simulink model "Basic_LogicGates"  (R2018a)
settings: Solver=VariableStepAuto  StartTime=0.0  StopTime=10.0  RelTol=1e-3
settings Model: Creator=Asus  LastModifiedBy=Asus

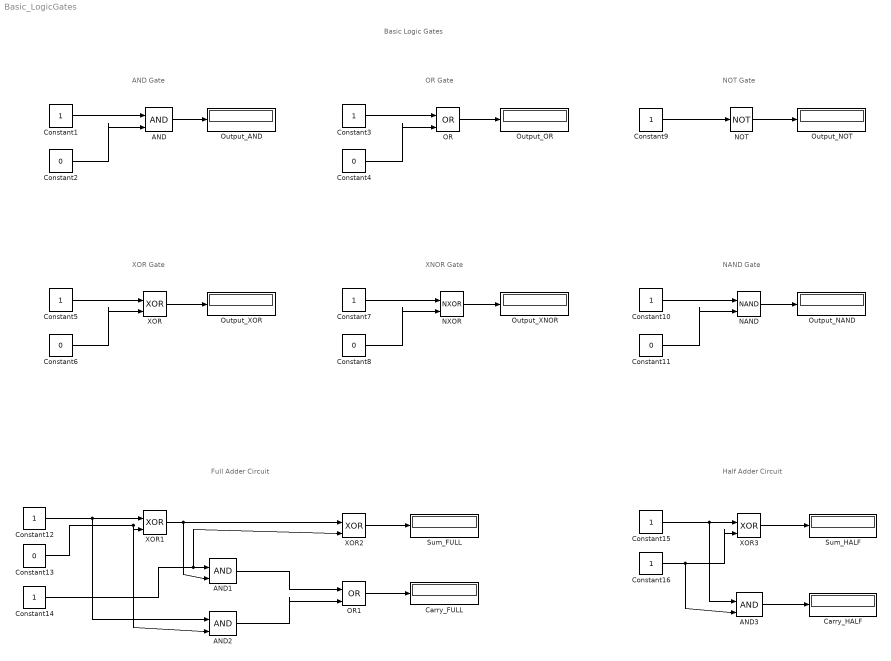
== system Basic_LogicGates ==
  note: Basic Logic Gates
  note: AND Gate
  note: OR Gate
  note: XOR Gate
  note: XNOR Gate
  note: NOT Gate
  note: NAND Gate
  note: Full Adder Circuit
  note: Half Adder Circuit
  AND{,1..3} (4 alike) : Logic  IconShape=distinctive  AllPortsSameDT=off  OutDataTypeStr=boolean
  Carry_FULL : Display
  Carry_HALF : Display
  Constant{1,3,5,7,9..10,12,14..16} (10 alike) : Constant
  Constant{2,4,6,8,11,13} (6 alike) : Constant  Value=0
  NAND : Logic  Operator=NAND  IconShape=distinctive  AllPortsSameDT=off  OutDataTypeStr=boolean
  NOT : Logic  Operator=NOT  IconShape=distinctive  AllPortsSameDT=off  OutDataTypeStr=boolean
  NXOR : Logic  Operator=NXOR  IconShape=distinctive  AllPortsSameDT=off  OutDataTypeStr=boolean
  OR : Logic  Operator=OR  IconShape=distinctive  AllPortsSameDT=off  OutDataTypeStr=boolean
  OR1 : Logic  Operator=OR  IconShape=distinctive  AllPortsSameDT=off  OutDataTypeStr=boolean
  Output_AND : Display
  Output_NAND : Display
  Output_NOT : Display
  Output_OR : Display
  Output_XNOR : Display
  Output_XOR : Display
  Sum_FULL : Display
  Sum_HALF : Display
  XOR{,1..3} (4 alike) : Logic  Operator=XOR  IconShape=distinctive  AllPortsSameDT=off  OutDataTypeStr=boolean
  wires:
  Constant1/1 -> AND/1
  Constant2/1 -> AND/2
  AND/1 -> Output_AND/1
  Constant4/1 -> OR/2
  Constant3/1 -> OR/1
  OR/1 -> Output_OR/1
  XOR/1 -> Output_XOR/1
  Constant5/1 -> XOR/1
  Constant6/1 -> XOR/2
  Constant8/1 -> NXOR/2
  Constant7/1 -> NXOR/1
  NXOR/1 -> Output_XNOR/1
  NOT/1 -> Output_NOT/1
  Constant9/1 -> NOT/1
  NAND/1 -> Output_NAND/1
  Constant10/1 -> NAND/1
  Constant11/1 -> NAND/2
  Constant12/1 -> AND2/1, XOR1/1
  XOR1/1 -> AND1/2, XOR2/1
  Constant13/1 -> AND2/2, XOR1/2
  Constant14/1 -> XOR2/2, AND1/1
  AND1/1 -> OR1/1
  AND2/1 -> OR1/2
  XOR2/1 -> Sum_FULL/1
  OR1/1 -> Carry_FULL/1
  Constant15/1 -> AND3/1, XOR3/1
  Constant16/1 -> AND3/2, XOR3/2
  XOR3/1 -> Sum_HALF/1
  AND3/1 -> Carry_HALF/1
